simulink library "isi_correlator_lib"  (Simulink 7.3)
settings: Solver=ode45  SolverMode=SingleTasking  StartTime=0.0  StopTime=10.0  RelTol=1e-3
libraries: xbsIndex_r4 x337, casper_library x37, xps_library x31, isi_correlator_lib x28
(part 1 of 3)
settings Model: Creator=wjm  LastModifiedBy=wjm

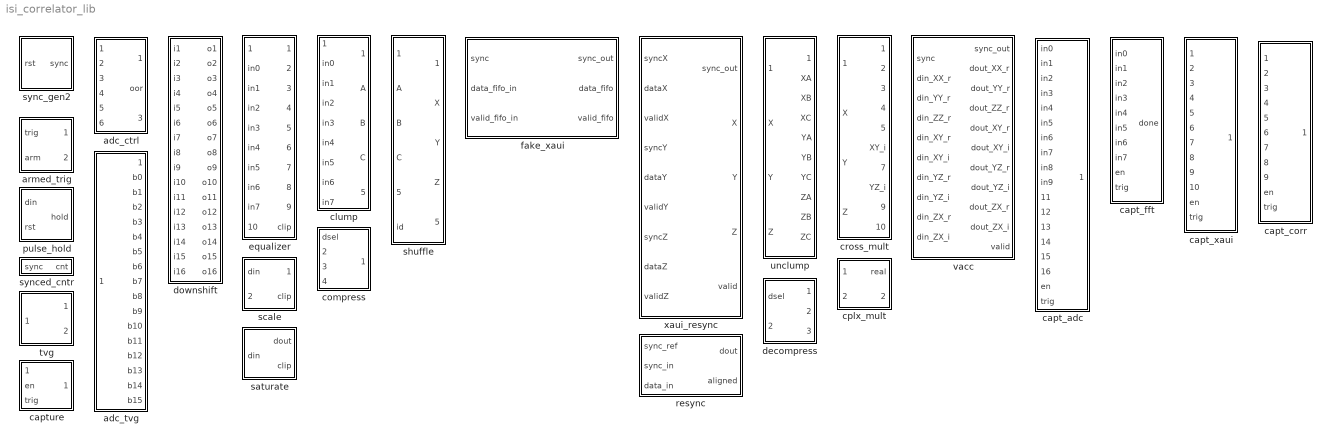
== system isi_correlator_lib ==
  adc_ctrl : Subsystem
  adc_tvg : Subsystem
  armed_trig : Subsystem
  capt_adc : Subsystem
  capt_corr : Subsystem
  capt_fft : Subsystem  mask{bit_width=18}
      mask prompts: bit_width "Bit width:"
  capt_xaui : Subsystem
  capture : Subsystem  mask(capture){num_brams=1, addr_width=11, done_port=off}
      mask prompts: num_brams "Number of BRAMs:"; addr_width "Address width:"; done_port "Provide done port"
      mask help: This block captures N data lines into N separate BRAMs.
      mask init:
      | capture_init(gcb, ...
      |     'num_brams', num_brams, ...
      |     'addr_width', addr_width, ...
      |     'done_port', done_port);
  clump : Subsystem  mask{latency=1}
  compress : Subsystem  mask{latency=1}
  cplx_mult : Subsystem  mask{in_bit_width=4, in_bin_point=3, mult_latency=3, add_latency=2}
      mask prompts: in_bit_width "Input bit width:"; in_bin_point "Input binary point:"; mult_latency "Mult latency:"; add_latency "Add latency:"
  cross_mult : Subsystem  mask{in_bit_width=4, in_bin_point=3, out_bit_width=8, out_bin_point=6, mult_latency=3, add_latency=2}
      mask prompts: in_bit_width "Input bit width: (cplx)"; in_bin_point "Input binary point: (cplx)"; out_bit_width "Output bit width: (cplx)"; out_bin_point "Output binary point: (cplx)"; mult_latency "Mult latency:"; add_latency "Add latency:"
  decompress : Subsystem  mask{latency=1}
  downshift : Subsystem  mask{bit_width=18}
      mask prompts: bit_width "Bit width:"
  equalizer : Subsystem  mask{in_bit_width=18, in_bin_point=17, coeff_bit_width=16, coeff_bin_point=8, out_bit_width=4, out_bin_point=3}
      mask prompts: in_bit_width "Input bit width:"; in_bin_point "Input binary point:"; coeff_bit_width "Coeff bit width:"; coeff_bin_point "Coeff binary point:"; out_bit_width "Output bit width:"; out_bin_point "Output binary point:"
  fake_xaui : Subsystem  mask{latency=64}
  pulse_hold : Subsystem
  resync : Subsystem  mask{depth=4}
      mask prompts: depth "Buffer depth: (2^?)"
  saturate : Subsystem  mask{in_bit_width=34, in_bin_point=25, out_bit_width=4, out_bin_point=3}
      mask prompts: in_bit_width "Input bit width:"; in_bin_point "Input binary point:"; out_bit_width "Output bit width:"; out_bin_point "Output binary point:"
  scale : Subsystem  mask{in_bit_width=8, in_bin_point=7, coeff_bit_width=16, coeff_bin_point=8, out_bit_width=5, out_bin_point=4}
      mask prompts: in_bit_width "Input bit width:"; in_bin_point "Input binary point:"; coeff_bit_width "Coeff bit width:"; coeff_bin_point "Coeff binary point:"; out_bit_width "Output bit width:"; out_bin_point "Output binary point:"
  shuffle : Subsystem  mask{latency=3}
  sync_gen2 : Subsystem  mask(sync_gen2){using_pfb_fir=off, pfb_fir_taps=1, using_fft=on, fft_size=7, fft_inputs=4, fft_orders=1, using_ct=off, ct_type=Double-buffered, using_vacc=off, vacc_length=0, using_scale_factor=off, scale_factor=1}
      mask prompts: using_pfb_fir "This design uses a PFB FIR."; pfb_fir_taps "Number of taps in PFB FIR:"; using_fft "This design uses an FFT."; fft_size "Size of FFT: (2^?)"; fft_inputs "Number of FFT inputs: (2^?)"; fft_orders "Order of FFT reorders: (vector)"; using_ct "This design uses a corner turner."; ct_type "Type of reorder operation:"; using_vacc "This design uses a vector accumulator."; vacc_length "Length of accumulations: (2^?)"; using_scale_factor "Scale the minimum period by an arbitrary amount."; scale_factor "Scale factor:"
      mask help: This block generates a sync pulse of an appropriate period based on the specified mask parameters.
      mask init:
      | sync_gen2_init(gcb, ...
      |     'using_pfb_fir', using_pfb_fir, ...
      |     'pfb_fir_taps', pfb_fir_taps, ...
      |     'using_fft', using_fft, ...
      |     'fft_size', fft_size, ...
      |     'fft_inputs', fft_inputs, ...
      |     'fft_orders', fft_orders, ...
      |     'using_ct', using_ct, ...
      |     'ct_type', ct_type, ...
      |     'using_vacc', using_vacc, ...
      |     'vacc_length', vacc_length, ...
      |     'using_scale_factor', using_scale_factor, ...
      |     'scale_factor', scale_factor);
      settings: AttributesFormatString=sync_period=8
      mask StyleString: checkbox,edit,checkbox,edit,edit,edit,checkbox,popup(Double-buffered|In-place),checkbox,edit,checkbox,edit
      mask CallbackString:
      | thisVariable = 'using_pfb_fir';
      | affectedVars = {'pfb_fir_taps'};
      | 
      | thisBlock = gcb();
      | thisVarState = get_param(thisBlock, thisVariable);
      | maskNames = get_param(thisBlock, 'MaskNames');
      | maskEnables = get_param(thisBlock, 'MaskEnables');
      | 
      | for varName = affectedVars
      |     varIndex = find(ismember(maskNames, varName));
      |     maskEnables{varIndex} = thisVarState;
      | end
      | 
      | set_param(thisBlock, 'MaskEnables', maskEnables);||thisVariable = 'using_fft';
      | affectedVars = {'fft_size', 'fft_inputs', 'fft_orders'};
      | 
      | thisBlock = gcb();
      | thisVarState = get_param(thisBlock, thisVariable);
      | maskNames = get_param(thisBlock, 'MaskNames');
      | maskEnables = get_param(thisBlock, 'MaskEnables');
      | 
      | for varName = affectedVars
      |     varIndex = find(ismember(maskNames, varName));
      |     maskEnables{varIndex} = thisVarState;
      | end
      | 
      | set_param(thisBlock, 'MaskEnables', maskEnables);||||thisVariable = 'using_ct';
      | affectedVars = {'ct_type'};
      | 
      | thisBlock = gcb();
      | thisVarState = get_param(thisBlock, thisVariable);
      | maskNames = get_param(thisBlock, 'MaskNames');
      | maskEnables = get_param(thisBlock, 'MaskEnables');
      | 
      | for varName = affectedVars
      |     varIndex = find(ismember(maskNames, varName));
      |     maskEnables{varIndex} = thisVarState;
      | end
      | 
      | set_param(thisBlock, 'MaskEnables', maskEnables);||thisVariable = 'using_vacc';
      | affectedVars = {'vacc_length'};
      | 
      | thisBlock = gcb();
      | thisVarState = get_param(thisBlock, thisVariable);
      | maskNames = get_param(thisBlock, 'MaskNames');
      | maskEnables = get_param(thisBlock, 'MaskEnables');
      | 
      | for varName = affectedVars
      |     varIndex = find(ismember(maskNames, varName));
      |     maskEnables{varIndex} = thisVarState;
      | end
      | 
      | set_param(thisBlock, 'MaskEnables', maskEnables);||thisVariable = 'using_scale_factor';
      | affectedVars = {'scale_factor'};
      | 
      | thisBlock = gcb();
      | thisVarState = get_param(thisBlock, thisVariable);
      | maskNames = get_param(thisBlock, 'MaskNames');
      | maskEnables = get_param(thisBlock, 'MaskEnables');
      | 
      | for varName = affectedVars
      |     varIndex = find(ismember(maskNames, varName));
      |     maskEnables{varIndex} = thisVarState;
      | end
      | 
      | set_param(thisBlock, 'MaskEnables', maskEnables);|
  synced_cntr : Subsystem  mask{bitwidth=2}
      mask prompts: bitwidth "Counter bitwidth:"
  tvg : Subsystem  mask{addr_width=11}
      mask prompts: addr_width "Address width:"
  unclump : Subsystem  mask{latency=1}
  vacc : Subsystem  mask{vector_length=8, out_bit_width=27, out_bin_point=4, and_delay=2}
      mask prompts: vector_length "Vector length:"; out_bit_width "Output bit width:"; out_bin_point "Output binary point:"; and_delay "Logic delay:"
  xaui_resync : Subsystem  mask(link_demux){buffer_depth=8, logic_latency=1}
      mask prompts: buffer_depth "Buffer depth: (2^n)"; logic_latency "Logic latency:"
      mask help: Demuxes three data streams from five links (one loopback and four xaui). Realigns the streams, and reconstructs a corresponding sync pulse.

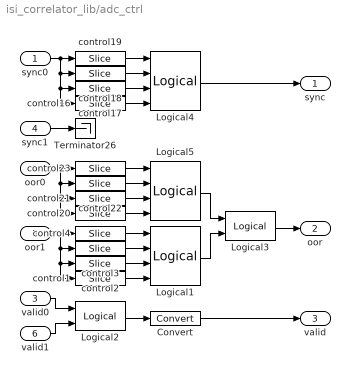
== system isi_correlator_lib/adc_ctrl ==
  sync0 : Inport  OutDataType=sfix(16)  OutScaling=2^0
  oor0 : Inport  Port=2  OutDataType=sfix(16)  OutScaling=2^0
  valid0 : Inport  Port=3  OutDataType=sfix(16)  OutScaling=2^0
  sync1 : Inport  Port=4  OutDataType=sfix(16)  OutScaling=2^0
  oor1 : Inport  Port=5  OutDataType=sfix(16)  OutScaling=2^0
  valid1 : Inport  Port=6  OutDataType=sfix(16)  OutScaling=2^0
  Convert : xbsIndex_r4/Convert  arith_type=Boolean  n_bits=1  bin_pt=0  quantization=Truncate  overflow=Wrap  latency=0  dbl_ovrd=off  pipeline=off  block_type=convert
      settings: block_version=11.3
  Logical1 : xbsIndex_r4/Logical  logical_function=OR  inputs=4  en=off  latency=0  precision=Full  arith_type=Unsigned  n_bits=1  bin_pt=0  align_bp=on  dbl_ovrd=off  block_type=logical
      settings: block_version=10.1.1
  Logical2 : xbsIndex_r4/Logical  logical_function=OR  inputs=2  en=off  latency=0  precision=Full  arith_type=Unsigned  n_bits=1  bin_pt=0  align_bp=on  dbl_ovrd=off  block_type=logical
      settings: block_version=10.1.1
  Logical3 : xbsIndex_r4/Logical  logical_function=OR  inputs=2  en=off  latency=0  precision=Full  arith_type=Unsigned  n_bits=1  bin_pt=0  align_bp=on  dbl_ovrd=off  block_type=logical
      settings: block_version=10.1.1
  Logical4 : xbsIndex_r4/Logical  logical_function=OR  inputs=4  en=off  latency=0  precision=Full  arith_type=Unsigned  n_bits=1  bin_pt=0  align_bp=on  dbl_ovrd=off  block_type=logical
      settings: block_version=10.1.1
  Logical5 : xbsIndex_r4/Logical  logical_function=OR  inputs=4  en=off  latency=0  precision=Full  arith_type=Unsigned  n_bits=1  bin_pt=0  align_bp=on  dbl_ovrd=off  block_type=logical
      settings: block_version=10.1.1
  Terminator26 : Terminator
  control1 : xbsIndex_r4/Slice  nbits=1  boolean_output=on  mode=Lower Bit Location + Width  bit1=0  base1=MSB of Input  bit0=0  base0=LSB of Input  dbl_ovrd=off  block_type=slice
      settings: block_version=10.1.3
  control16 : xbsIndex_r4/Slice  nbits=1  boolean_output=on  mode=Lower Bit Location + Width  bit1=0  base1=MSB of Input  bit0=0  base0=LSB of Input  dbl_ovrd=off  block_type=slice
      settings: block_version=10.1.3
  control17 : xbsIndex_r4/Slice  nbits=1  boolean_output=on  mode=Lower Bit Location + Width  bit1=0  base1=MSB of Input  bit0=1  base0=LSB of Input  dbl_ovrd=off  block_type=slice
      settings: block_version=10.1.3
  control18 : xbsIndex_r4/Slice  nbits=1  boolean_output=on  mode=Lower Bit Location + Width  bit1=0  base1=MSB of Input  bit0=2  base0=LSB of Input  dbl_ovrd=off  block_type=slice
      settings: block_version=10.1.3
  control19 : xbsIndex_r4/Slice  nbits=1  boolean_output=on  mode=Lower Bit Location + Width  bit1=0  base1=MSB of Input  bit0=3  base0=LSB of Input  dbl_ovrd=off  block_type=slice
      settings: block_version=10.1.3
  control2 : xbsIndex_r4/Slice  nbits=1  boolean_output=on  mode=Lower Bit Location + Width  bit1=0  base1=MSB of Input  bit0=1  base0=LSB of Input  dbl_ovrd=off  block_type=slice
      settings: block_version=10.1.3
  control20 : xbsIndex_r4/Slice  nbits=1  boolean_output=on  mode=Lower Bit Location + Width  bit1=0  base1=MSB of Input  bit0=0  base0=LSB of Input  dbl_ovrd=off  block_type=slice
      settings: block_version=10.1.3
  control21 : xbsIndex_r4/Slice  nbits=1  boolean_output=on  mode=Lower Bit Location + Width  bit1=0  base1=MSB of Input  bit0=1  base0=LSB of Input  dbl_ovrd=off  block_type=slice
      settings: block_version=10.1.3
  control22 : xbsIndex_r4/Slice  nbits=1  boolean_output=on  mode=Lower Bit Location + Width  bit1=0  base1=MSB of Input  bit0=2  base0=LSB of Input  dbl_ovrd=off  block_type=slice
      settings: block_version=10.1.3
  control23 : xbsIndex_r4/Slice  nbits=1  boolean_output=on  mode=Lower Bit Location + Width  bit1=0  base1=MSB of Input  bit0=3  base0=LSB of Input  dbl_ovrd=off  block_type=slice
      settings: block_version=10.1.3
  control3 : xbsIndex_r4/Slice  nbits=1  boolean_output=on  mode=Lower Bit Location + Width  bit1=0  base1=MSB of Input  bit0=2  base0=LSB of Input  dbl_ovrd=off  block_type=slice
      settings: block_version=10.1.3
  control4 : xbsIndex_r4/Slice  nbits=1  boolean_output=on  mode=Lower Bit Location + Width  bit1=0  base1=MSB of Input  bit0=3  base0=LSB of Input  dbl_ovrd=off  block_type=slice
      settings: block_version=10.1.3
  sync : Outport  OutDataType=sfix(16)  OutScaling=2^0
  oor : Outport  Port=2  OutDataType=sfix(16)  OutScaling=2^0
  valid : Outport  Port=3  OutDataType=sfix(16)  OutScaling=2^0
  wires:
  Logical2/1 -> Convert/1
  Convert/1 -> valid/1
  control23/1 -> Logical5/1
  control22/1 -> Logical5/2
  control21/1 -> Logical5/3
  control20/1 -> Logical5/4
  sync0/1 -> control19/1, control18/1, control16/1, control17/1
  control19/1 -> Logical4/1
  control18/1 -> Logical4/2
  control17/1 -> Logical4/3
  control16/1 -> Logical4/4
  oor0/1 -> control23/1, control22/1, control20/1, control21/1
  control4/1 -> Logical1/1
  control3/1 -> Logical1/2
  control2/1 -> Logical1/3
  control1/1 -> Logical1/4
  Logical5/1 -> Logical3/1
  Logical1/1 -> Logical3/2
  sync1/1 -> Terminator26/1
  Logical3/1 -> oor/1
  Logical4/1 -> sync/1
  oor1/1 -> control4/1, control3/1, control1/1, control2/1
  valid0/1 -> Logical2/1
  valid1/1 -> Logical2/2

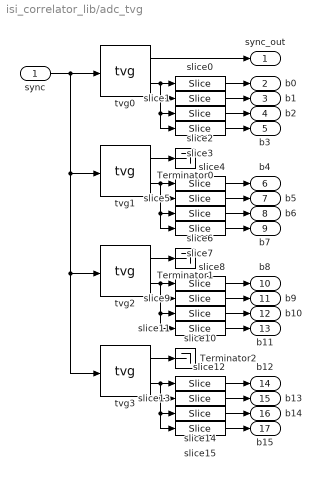
== system isi_correlator_lib/adc_tvg ==
  sync : Inport  OutDataType=sfix(16)  OutScaling=2^0
  Terminator0 : Terminator
  Terminator1 : Terminator
  Terminator2 : Terminator
  slice{0,4,8,12} (4 alike) : xbsIndex_r4/Slice  nbits=8  boolean_output=off  mode=Lower Bit Location + Width  bit1=0  base1=MSB of Input  bit0=0  base0=LSB of Input  dbl_ovrd=off  block_type=slice
      settings: block_version=10.1.3
  slice{1,5,9,13} (4 alike) : xbsIndex_r4/Slice  nbits=8  boolean_output=off  mode=Lower Bit Location + Width  bit1=0  base1=MSB of Input  bit0=8  base0=LSB of Input  dbl_ovrd=off  block_type=slice
      settings: block_version=10.1.3
  slice{2,6,10,14} (4 alike) : xbsIndex_r4/Slice  nbits=8  boolean_output=off  mode=Lower Bit Location + Width  bit1=0  base1=MSB of Input  bit0=16  base0=LSB of Input  dbl_ovrd=off  block_type=slice
      settings: block_version=10.1.3
  slice{3,7,11,15} (4 alike) : xbsIndex_r4/Slice  nbits=8  boolean_output=off  mode=Lower Bit Location + Width  bit1=0  base1=MSB of Input  bit0=24  base0=LSB of Input  dbl_ovrd=off  block_type=slice
      settings: block_version=10.1.3
  tvg{0..3} (4 alike) : isi_correlator_lib/tvg  SystemSampleTime=-1  addr_width=11
  sync_out : Outport
  b0 : Outport  Port=2
  b1 : Outport  Port=3
  b2 : Outport  Port=4
  b3 : Outport  Port=5
  b4 : Outport  Port=6
  b5 : Outport  Port=7
  b6 : Outport  Port=8
  b7 : Outport  Port=9
  b8 : Outport  Port=10
  b9 : Outport  Port=11
  b10 : Outport  Port=12
  b11 : Outport  Port=13
  b12 : Outport  Port=14
  b13 : Outport  Port=15
  b14 : Outport  Port=16
  b15 : Outport  Port=17
  wires:
  tvg3/2 -> slice14/1, slice15/1, slice13/1, slice12/1
  tvg2/2 -> slice10/1, slice11/1, slice9/1, slice8/1
  tvg1/2 -> slice6/1, slice7/1, slice5/1, slice4/1
  tvg0/2 -> slice2/1, slice3/1, slice1/1, slice0/1
  tvg0/1 -> sync_out/1
  slice0/1 -> b0/1
  slice1/1 -> b1/1
  slice2/1 -> b2/1
  slice3/1 -> b3/1
  slice4/1 -> b4/1
  slice5/1 -> b5/1
  slice6/1 -> b6/1
  slice7/1 -> b7/1
  slice8/1 -> b8/1
  slice9/1 -> b9/1
  slice10/1 -> b10/1
  slice11/1 -> b11/1
  slice12/1 -> b12/1
  slice13/1 -> b13/1
  slice14/1 -> b14/1
  slice15/1 -> b15/1
  sync/1 -> tvg0/1, tvg1/1, tvg3/1, tvg2/1
  tvg1/1 -> Terminator0/1
  tvg2/1 -> Terminator1/1
  tvg3/1 -> Terminator2/1

== system isi_correlator_lib/armed_trig ==
  trig : Inport  OutDataType=sfix(16)  OutScaling=2^0
  arm : Inport  Port=2  OutDataType=sfix(16)  OutScaling=2^0
  Constant : xbsIndex_r4/Constant  arith_type=Boolean  const=1  n_bits=1  bin_pt=0  explicit_period=on  period=1  equ=P=C  opselect=C  inp2=PCIN>>17  opr=+  inp1=P  carry=CIN  dbl_ovrd=off  block_type=constant
  Logical : xbsIndex_r4/Logical  logical_function=AND  inputs=2  en=off  latency=0  precision=Full  arith_type=Unsigned  n_bits=16  bin_pt=0  align_bp=on  dbl_ovrd=off  block_type=logical
  Register : xbsIndex_r4/Register  init=0  rst=on  en=on  dbl_ovrd=off  block_type=register
  posedge : casper_library/Misc/posedge  Tag=Rising Edge Detector  SystemSampleTime=-1
  trig_out : Outport  OutDataType=sfix(16)  OutScaling=2^0
  armed : Outport  Port=2  OutDataType=sfix(16)  OutScaling=2^0
  wires:
  trig/1 -> Logical/1
  Register/1 -> Logical/2, armed/1
  arm/1 -> posedge/1
  Constant/1 -> Register/1
  posedge/1 -> Register/3
  Logical/1 -> trig_out/1, Register/2

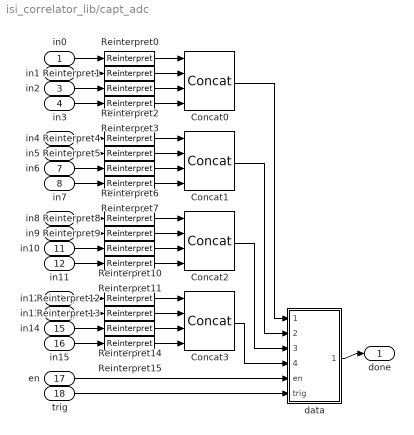
== system isi_correlator_lib/capt_adc ==
  in0 : Inport
  in1 : Inport  Port=2
  in2 : Inport  Port=3
  in3 : Inport  Port=4
  in4 : Inport  Port=5
  in5 : Inport  Port=6
  in6 : Inport  Port=7
  in7 : Inport  Port=8
  in8 : Inport  Port=9
  in9 : Inport  Port=10
  in10 : Inport  Port=11
  in11 : Inport  Port=12
  in12 : Inport  Port=13
  in13 : Inport  Port=14
  in14 : Inport  Port=15
  in15 : Inport  Port=16
  en : Inport  Port=17
  trig : Inport  Port=18
  Concat{0..3} (4 alike) : xbsIndex_r4/Concat  num_inputs=4  dbl_ovrd=off  block_type=concat
      settings: block_version=10.1.3
  Reinterpret{0..15} (16 alike) : xbsIndex_r4/Reinterpret  force_arith_type=on  arith_type=Unsigned  force_bin_pt=on  bin_pt=0  block_type=reinterpret
      settings: infoedit="Changes signal type without altering the binary representation.   You can changed the signal between signed and unsigned, and relocate the binary point.<P><P>Hardware notes: In hardware this block costs nothing.<P><P>Example:  Suppose the input is 6 bits wide, signed, with 2 fractional bits, and the output is forced to unsigned with 0 fractional bits.  Then an input of -2.0 (1110.00 in binary 2's complement) becomes an output of 56 (111000 in binary)."  block_version=10.1.3
  data : Subsystem  AncestorBlock=isi_correlator_lib/capture  mask(capture){num_brams=4, addr_width=11, done_port=on}
      mask prompts: num_brams "Number of BRAMs:"; addr_width "Address width:"; done_port "Provide done port"
      mask help: This block captures N data lines into N separate BRAMs.
      mask init:
      | capture_init(gcb, ...
      |     'num_brams', num_brams, ...
      |     'addr_width', addr_width, ...
      |     'done_port', done_port);
  done : Outport
  wires:
  Concat3/1 -> data/4(din3)
  Concat2/1 -> data/3(din2)
  Concat1/1 -> data/2(din1)
  Concat0/1 -> data/1(din0)
  trig/1 -> data/6(trig)
  en/1 -> data/5(en)
  Reinterpret15/1 -> Concat3/4
  Reinterpret14/1 -> Concat3/3
  Reinterpret13/1 -> Concat3/2
  Reinterpret12/1 -> Concat3/1
  Reinterpret11/1 -> Concat2/4
  Reinterpret10/1 -> Concat2/3
  Reinterpret9/1 -> Concat2/2
  Reinterpret8/1 -> Concat2/1
  Reinterpret7/1 -> Concat1/4
  Reinterpret6/1 -> Concat1/3
  Reinterpret5/1 -> Concat1/2
  Reinterpret4/1 -> Concat1/1
  Reinterpret3/1 -> Concat0/4
  Reinterpret2/1 -> Concat0/3
  Reinterpret1/1 -> Concat0/2
  Reinterpret0/1 -> Concat0/1
  in0/1 -> Reinterpret0/1
  in1/1 -> Reinterpret1/1
  in2/1 -> Reinterpret2/1
  in3/1 -> Reinterpret3/1
  in4/1 -> Reinterpret4/1
  in5/1 -> Reinterpret5/1
  in6/1 -> Reinterpret6/1
  in7/1 -> Reinterpret7/1
  in8/1 -> Reinterpret8/1
  in9/1 -> Reinterpret9/1
  in10/1 -> Reinterpret10/1
  in11/1 -> Reinterpret11/1
  in12/1 -> Reinterpret12/1
  in13/1 -> Reinterpret13/1
  in14/1 -> Reinterpret14/1
  in15/1 -> Reinterpret15/1
  data/1(done) -> done/1

== system isi_correlator_lib/capt_corr ==
  AA_r : Inport
  BB_r : Inport  Port=2
  CC_r : Inport  Port=3
  AB_r : Inport  Port=4
  AB_i : Inport  Port=5
  BC_r : Inport  Port=6
  BC_i : Inport  Port=7
  CA_r : Inport  Port=8
  CA_i : Inport  Port=9
  en : Inport  Port=10
  trig : Inport  Port=11
  capt0 : Subsystem  AncestorBlock=isi_correlator_lib/capture  mask(capture){num_brams=3, addr_width=11, done_port=off}
      mask prompts: num_brams "Number of BRAMs:"; addr_width "Address width:"; done_port "Provide done port"
      mask help: This block captures N data lines into N separate BRAMs.
      mask init:
      | capture_init(gcb, ...
      |     'num_brams', num_brams, ...
      |     'addr_width', addr_width, ...
      |     'done_port', done_port);
  capt1 : Subsystem  AncestorBlock=isi_correlator_lib/capture  mask(capture){num_brams=3, addr_width=11, done_port=off}
      mask prompts: num_brams "Number of BRAMs:"; addr_width "Address width:"; done_port "Provide done port"
      mask help: This block captures N data lines into N separate BRAMs.
      mask init:
      | capture_init(gcb, ...
      |     'num_brams', num_brams, ...
      |     'addr_width', addr_width, ...
      |     'done_port', done_port);
  capt2 : Subsystem  AncestorBlock=isi_correlator_lib/capture  mask(capture){num_brams=3, addr_width=11, done_port=off}
      mask prompts: num_brams "Number of BRAMs:"; addr_width "Address width:"; done_port "Provide done port"
      mask help: This block captures N data lines into N separate BRAMs.
      mask init:
      | capture_init(gcb, ...
      |     'num_brams', num_brams, ...
      |     'addr_width', addr_width, ...
      |     'done_port', done_port);
  done : Outport
  wires:
  AA_r/1 -> capt0/1(din0)
  BB_r/1 -> capt0/2(din1)
  CC_r/1 -> capt0/3(din2)
  AB_r/1 -> capt1/1(din0)
  AB_i/1 -> capt1/2(din1)
  BC_r/1 -> capt1/3(din2)
  BC_i/1 -> capt2/1(din0)
  CA_r/1 -> capt2/2(din1)
  CA_i/1 -> capt2/3(din2)
  en/1 -> capt2/4(en), capt0/4(en), capt1/4(en)
  trig/1 -> capt2/5(trig), capt0/5(trig), capt1/5(trig)
  capt0/1(done) -> done/1

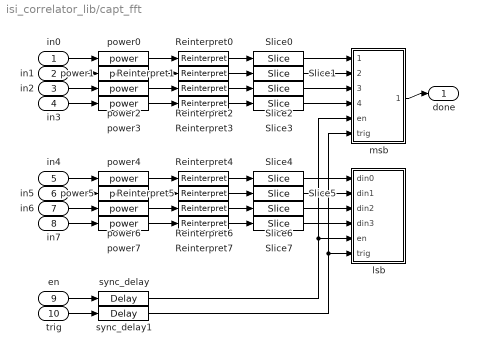
== system isi_correlator_lib/capt_fft ==
  in0 : Inport
  in1 : Inport  Port=2
  in2 : Inport  Port=3
  in3 : Inport  Port=4
  in4 : Inport  Port=5
  in5 : Inport  Port=6
  in6 : Inport  Port=7
  in7 : Inport  Port=8
  en : Inport  Port=9
  trig : Inport  Port=10
  Reinterpret{0..7} (8 alike) : xbsIndex_r4/Reinterpret  force_arith_type=on  arith_type=Unsigned  force_bin_pt=on  bin_pt=0  block_type=reinterpret
      settings: infoedit="Changes signal type without altering the binary representation.   You can changed the signal between signed and unsigned, and relocate the binary point.<P><P>Hardware notes: In hardware this block costs nothing.<P><P>Example:  Suppose the input is 6 bits wide, signed, with 2 fractional bits, and the output is forced to unsigned with 0 fractional bits.  Then an input of -2.0 (1110.00 in binary 2's complement) becomes an output of 56 (111000 in binary)."  block_version=10.1.3
  Slice{0..7} (8 alike) : xbsIndex_r4/Slice  nbits=min(32, bit_width*2)  boolean_output=off  mode=Upper Bit Location + Width  bit1=0  base1=MSB of Input  bit0=0  base0=LSB of Input  dbl_ovrd=off  block_type=slice
      settings: block_version=11.3
  lsb : Subsystem  AncestorBlock=isi_correlator_lib/capture  mask(capture){num_brams=4, addr_width=11, done_port=off}
      mask prompts: num_brams "Number of BRAMs:"; addr_width "Address width:"; done_port "Provide done port"
      mask help: This block captures N data lines into N separate BRAMs.
      mask init:
      | capture_init(gcb, ...
      |     'num_brams', num_brams, ...
      |     'addr_width', addr_width, ...
      |     'done_port', done_port);
  msb : Subsystem  AncestorBlock=isi_correlator_lib/capture  mask(capture){num_brams=4, addr_width=11, done_port=off}
      mask prompts: num_brams "Number of BRAMs:"; addr_width "Address width:"; done_port "Provide done port"
      mask help: This block captures N data lines into N separate BRAMs.
      mask init:
      | capture_init(gcb, ...
      |     'num_brams', num_brams, ...
      |     'addr_width', addr_width, ...
      |     'done_port', done_port);
  power{0..7} (8 alike) : casper_library/Misc/power  SystemSampleTime=-1  BitWidth=bit_width  add_latency=2  mult_latency=3
  sync_delay : xbsIndex_r4/Delay  en=off  latency=5  dbl_ovrd=off  reg_retiming=off  block_type=delay
  sync_delay1 : xbsIndex_r4/Delay  en=off  latency=5  dbl_ovrd=off  reg_retiming=off  block_type=delay
  done : Outport
  wires:
  power7/1 -> Reinterpret7/1
  in7/1 -> power7/1
  trig/1 -> sync_delay1/1
  en/1 -> sync_delay/1
  Reinterpret3/1 -> Slice3/1
  Reinterpret2/1 -> Slice2/1
  Reinterpret1/1 -> Slice1/1
  Reinterpret7/1 -> Slice7/1
  Reinterpret6/1 -> Slice6/1
  Reinterpret5/1 -> Slice5/1
  Reinterpret4/1 -> Slice4/1
  power6/1 -> Reinterpret6/1
  in6/1 -> power6/1
  power5/1 -> Reinterpret5/1
  in5/1 -> power5/1
  power4/1 -> Reinterpret4/1
  in4/1 -> power4/1
  power3/1 -> Reinterpret3/1
  in3/1 -> power3/1
  power2/1 -> Reinterpret2/1
  in2/1 -> power2/1
  power1/1 -> Reinterpret1/1
  in1/1 -> power1/1
  Reinterpret0/1 -> Slice0/1
  power0/1 -> Reinterpret0/1
  in0/1 -> power0/1
  sync_delay/1 -> msb/5(en), lsb/5(en)
  sync_delay1/1 -> msb/6(trig), lsb/6(trig)
  Slice0/1 -> msb/1(din0)
  Slice1/1 -> msb/2(din1)
  Slice2/1 -> msb/3(din2)
  Slice3/1 -> msb/4(din3)
  Slice4/1 -> lsb/1(din0)
  Slice5/1 -> lsb/2(din1)
  Slice6/1 -> lsb/3(din2)
  Slice7/1 -> lsb/4(din3)
  msb/1(done) -> done/1

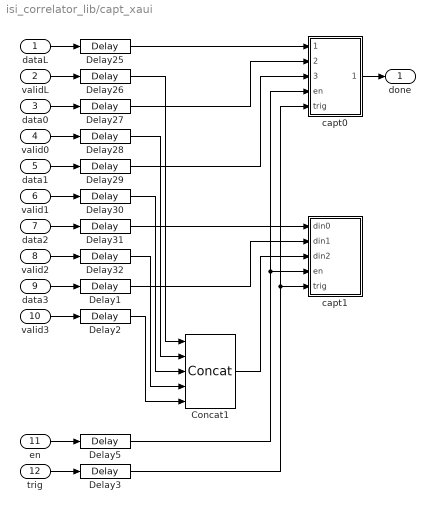
== system isi_correlator_lib/capt_xaui ==
  dataL : Inport
  validL : Inport  Port=2
  data0 : Inport  Port=3
  valid0 : Inport  Port=4
  data1 : Inport  Port=5
  valid1 : Inport  Port=6
  data2 : Inport  Port=7
  valid2 : Inport  Port=8
  data3 : Inport  Port=9
  valid3 : Inport  Port=10
  en : Inport  Port=11
  trig : Inport  Port=12
  Concat1 : xbsIndex_r4/Concat  num_inputs=5  dbl_ovrd=off  block_type=concat
      settings: block_version=10.1.3
  Delay{1..3,5,25..32} (12 alike) : xbsIndex_r4/Delay  en=off  latency=2  dbl_ovrd=off  reg_retiming=off  block_type=delay
  capt0 : Subsystem  AncestorBlock=isi_correlator_lib/capture  mask(capture){num_brams=3, addr_width=11, done_port=off}
      mask prompts: num_brams "Number of BRAMs:"; addr_width "Address width:"; done_port "Provide done port"
      mask help: This block captures N data lines into N separate BRAMs.
      mask init:
      | capture_init(gcb, ...
      |     'num_brams', num_brams, ...
      |     'addr_width', addr_width, ...
      |     'done_port', done_port);
  capt1 : Subsystem  AncestorBlock=isi_correlator_lib/capture  mask(capture){num_brams=3, addr_width=11, done_port=off}
      mask prompts: num_brams "Number of BRAMs:"; addr_width "Address width:"; done_port "Provide done port"
      mask help: This block captures N data lines into N separate BRAMs.
      mask init:
      | capture_init(gcb, ...
      |     'num_brams', num_brams, ...
      |     'addr_width', addr_width, ...
      |     'done_port', done_port);
  done : Outport
  wires:
  dataL/1 -> Delay25/1
  validL/1 -> Delay26/1
  data0/1 -> Delay27/1
  valid0/1 -> Delay28/1
  data1/1 -> Delay29/1
  valid1/1 -> Delay30/1
  data2/1 -> Delay31/1
  valid2/1 -> Delay32/1
  data3/1 -> Delay1/1
  valid3/1 -> Delay2/1
  Delay26/1 -> Concat1/1
  Delay28/1 -> Concat1/2
  Delay30/1 -> Concat1/3
  Delay32/1 -> Concat1/4
  Delay2/1 -> Concat1/5
  Delay31/1 -> capt1/1(din0)
  Delay1/1 -> capt1/2(din1)
  Concat1/1 -> capt1/3(din2)
  Delay25/1 -> capt0/1(din0)
  Delay27/1 -> capt0/2(din1)
  Delay29/1 -> capt0/3(din2)
  en/1 -> Delay5/1
  trig/1 -> Delay3/1
  Delay5/1 -> capt0/4(en), capt1/4(en)
  Delay3/1 -> capt0/5(trig), capt1/5(trig)
  capt0/1(done) -> done/1

== system isi_correlator_lib/capture ==
  din0 : Inport
  en : Inport  Port=2
  trig : Inport  Port=3
  Constant : xbsIndex_r4/Constant  arith_type=Boolean  const=1  n_bits=1  bin_pt=0  explicit_period=on  period=1  equ=P=C  opselect=C  inp2=PCIN>>17  opr=+  inp1=P  carry=CIN  dbl_ovrd=off  block_type=constant
      settings: block_version=11.3
  Logical : xbsIndex_r4/Logical  logical_function=AND  inputs=2  en=off  latency=0  precision=Full  arith_type=Unsigned  n_bits=16  bin_pt=0  align_bp=on  dbl_ovrd=off  block_type=logical
      settings: block_version=11.3
  bram0 : xps_library/Shared BRAM  Tag=xps:bram  SystemSampleTime=-1  arith_type=Unsigned  addr_width=addr_width  data_width=32  data_bin_pt=0  init_vals=0  sample_rate=1
  freeze_cntr : casper_library/Misc/freeze_cntr  SystemSampleTime=-1  CounterBits=addr_width
  reinterp0 : xbsIndex_r4/Reinterpret  force_arith_type=on  arith_type=Unsigned  force_bin_pt=on  bin_pt=0  block_type=reinterpret
      settings: infoedit="Changes signal type without altering the binary representation.   You can changed the signal between signed and unsigned, and relocate the binary point.<br><br>Hardware notes: In hardware this block costs nothing.<br><br>Example:  Suppose the input is 6 bits wide, signed, with 2 fractional bits, and the output is forced to unsigned with 0 fractional bits.  Then an input of -2.0 (1110.00 in binary 2's complement) becomes an output of 56 (111000 in binary)."  block_version=11.3
  terminator0 : Terminator
  done : Outport
  wires:
  din0/1 -> reinterp0/1
  reinterp0/1 -> bram0/2
  bram0/1 -> terminator0/1
  freeze_cntr/3 -> done/1
  en/1 -> Logical/1
  trig/1 -> Logical/2
  Constant/1 -> freeze_cntr/1
  Logical/1 -> freeze_cntr/2
  freeze_cntr/1 -> bram0/1
  freeze_cntr/2 -> bram0/3

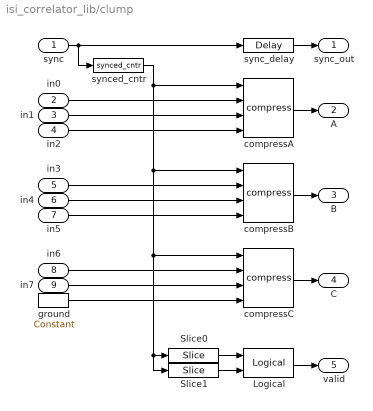
== system isi_correlator_lib/clump ==
  sync : Inport
  in0 : Inport  Port=2
  in1 : Inport  Port=3
  in2 : Inport  Port=4
  in3 : Inport  Port=5
  in4 : Inport  Port=6
  in5 : Inport  Port=7
  in6 : Inport  Port=8
  in7 : Inport  Port=9
  Logical : xbsIndex_r4/Logical  logical_function=OR  inputs=2  en=off  latency=latency  precision=Full  arith_type=Unsigned  n_bits=16  bin_pt=0  align_bp=on  dbl_ovrd=off  block_type=logical
  Slice0 : xbsIndex_r4/Slice  nbits=1  boolean_output=on  mode=Lower Bit Location + Width  bit1=0  base1=MSB of Input  bit0=0  base0=LSB of Input  dbl_ovrd=off  block_type=slice
      settings: block_version=10.1.1
  Slice1 : xbsIndex_r4/Slice  nbits=1  boolean_output=on  mode=Lower Bit Location + Width  bit1=0  base1=MSB of Input  bit0=1  base0=LSB of Input  dbl_ovrd=off  block_type=slice
      settings: block_version=10.1.1
  compressA : isi_correlator_lib/compress  SystemSampleTime=-1  latency=latency
  compressB : isi_correlator_lib/compress  SystemSampleTime=-1  latency=latency
  compressC : isi_correlator_lib/compress  SystemSampleTime=-1  latency=latency
  ground : xbsIndex_r4/Constant  arith_type=Unsigned  const=0  n_bits=8  bin_pt=0  explicit_period=on  period=1  equ=P=C  opselect=C  inp2=PCIN>>17  opr=+  inp1=P  carry=CIN  dbl_ovrd=off  block_type=constant
      settings: block_version=10.1.1
  sync_delay : xbsIndex_r4/Delay  en=off  latency=latency  dbl_ovrd=off  reg_retiming=off  block_type=delay
  synced_cntr : isi_correlator_lib/synced_cntr  SystemSampleTime=-1  bitwidth=2
  sync_out : Outport
  A : Outport  Port=2
  B : Outport  Port=3
  C : Outport  Port=4
  valid : Outport  Port=5
  wires:
  Slice0/1 -> Logical/1
  Slice1/1 -> Logical/2
  Logical/1 -> valid/1
  compressA/1 -> A/1
  compressB/1 -> B/1
  compressC/1 -> C/1
  sync_delay/1 -> sync_out/1
  sync/1 -> sync_delay/1, synced_cntr/1
  in3/1 -> compressB/2
  in4/1 -> compressB/3
  in5/1 -> compressB/4
  in6/1 -> compressC/2
  in7/1 -> compressC/3
  ground/1 -> compressC/4
  in0/1 -> compressA/2
  in1/1 -> compressA/3
  in2/1 -> compressA/4
  synced_cntr/1 -> Slice1/1, Slice0/1, compressC/1, compressB/1, compressA/1

== system isi_correlator_lib/compress ==
  dsel : Inport
  din0 : Inport  Port=2
  din1 : Inport  Port=3
  din2 : Inport  Port=4
  Concat0 : xbsIndex_r4/Concat  num_inputs=3  dbl_ovrd=off  block_type=concat
      settings: block_version=11.3
  Concat1 : xbsIndex_r4/Concat  num_inputs=2  dbl_ovrd=off  block_type=concat
      settings: block_version=11.3
  Constant : xbsIndex_r4/Constant  arith_type=Unsigned  const=0  n_bits=32  bin_pt=0  explicit_period=on  period=1  equ=P=C  opselect=C  inp2=PCIN>>17  opr=+  inp1=P  carry=CIN  dbl_ovrd=off  block_type=constant
      settings: block_version=11.3
  Delay0 : xbsIndex_r4/Delay  en=off  latency=1  dbl_ovrd=off  reg_retiming=off  block_type=delay
  Mux : xbsIndex_r4/Mux  inputs=4  en=off  latency=latency  precision=Full  arith_type=Unsigned  n_bits=16  bin_pt=14  quantization=Truncate  overflow=Wrap  dbl_ovrd=off  block_type=mux
  Slice0 : xbsIndex_r4/Slice  nbits=32  boolean_output=off  mode=Upper Bit Location + Width  bit1=0  base1=MSB of Input  bit0=0  base0=LSB of Input  dbl_ovrd=off  block_type=slice
      settings: block_version=10.1.1
  Slice1 : xbsIndex_r4/Slice  nbits=32  boolean_output=off  mode=Upper Bit Location + Width  bit1=-8  base1=MSB of Input  bit0=0  base0=LSB of Input  dbl_ovrd=off  block_type=slice
      settings: block_version=10.1.1
  Slice2 : xbsIndex_r4/Slice  nbits=32  boolean_output=off  mode=Upper Bit Location + Width  bit1=-16  base1=MSB of Input  bit0=0  base0=LSB of Input  dbl_ovrd=off  block_type=slice
      settings: block_version=10.1.1
  data : Outport
  wires:
  din0/1 -> Concat0/1
  din1/1 -> Concat0/2
  din2/1 -> Concat0/3
  Concat0/1 -> Delay0/1, Concat1/2
  Delay0/1 -> Concat1/1
  Concat1/1 -> Slice0/1, Slice2/1, Slice1/1
  dsel/1 -> Mux/1
  Mux/1 -> data/1
  Constant/1 -> Mux/2
  Slice0/1 -> Mux/3
  Slice1/1 -> Mux/4
  Slice2/1 -> Mux/5

== system isi_correlator_lib/cplx_mult ==
  a+bi : Inport  OutDataType=sfix(16)  OutScaling=2^0
  c+di : Inport  Port=2  OutDataType=sfix(16)  OutScaling=2^0
  c_to_ri : casper_library/Misc/c_to_ri  SystemSampleTime=-1  n_bits=in_bit_width  bin_pt=in_bin_point
      settings: AttributesFormatString=_ r/i
  c_to_ri1 : casper_library/Misc/c_to_ri  SystemSampleTime=-1  n_bits=in_bit_width  bin_pt=in_bin_point
      settings: AttributesFormatString=_ r/i
  cmult_4bit_em* : casper_library/Multipliers/cmult_4bit_em*  SystemSampleTime=-1  mult_latency=mult_latency  add_latency=add_latency
  real : Outport  OutDataType=sfix(16)  OutScaling=2^0
  imag : Outport  Port=2  OutDataType=sfix(16)  OutScaling=2^0
  wires:
  c_to_ri/1 -> cmult_4bit_em*/1
  c_to_ri/2 -> cmult_4bit_em*/2
  c_to_ri1/1 -> cmult_4bit_em*/3
  c_to_ri1/2 -> cmult_4bit_em*/4
  a+bi/1 -> c_to_ri/1
  c+di/1 -> c_to_ri1/1
  cmult_4bit_em*/1 -> real/1
  cmult_4bit_em*/2 -> imag/1

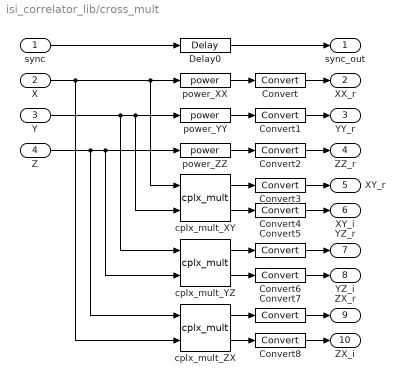
== system isi_correlator_lib/cross_mult ==
  sync : Inport  OutDataType=sfix(16)  OutScaling=2^0
  X : Inport  Port=2  OutDataType=sfix(16)  OutScaling=2^0
  Y : Inport  Port=3  OutDataType=sfix(16)  OutScaling=2^0
  Z : Inport  Port=4  OutDataType=sfix(16)  OutScaling=2^0
  Convert{,1..8} (9 alike) : xbsIndex_r4/Convert  arith_type="Signed  (2's comp)"  n_bits=out_bit_width  bin_pt=out_bin_point  quantization=Truncate  overflow=Wrap  latency=0  dbl_ovrd=off  pipeline=off  block_type=convert
      settings: block_version=10.1.3
  Delay0 : xbsIndex_r4/Delay  en=off  latency=mult_latency + add_latency  dbl_ovrd=off  reg_retiming=off  block_type=delay
  cplx_mult_XY : isi_correlator_lib/cplx_mult  SystemSampleTime=-1  in_bit_width=in_bit_width  in_bin_point=in_bin_point  mult_latency=mult_latency  add_latency=add_latency
  cplx_mult_YZ : isi_correlator_lib/cplx_mult  SystemSampleTime=-1  in_bit_width=in_bit_width  in_bin_point=in_bin_point  mult_latency=mult_latency  add_latency=add_latency
  cplx_mult_ZX : isi_correlator_lib/cplx_mult  SystemSampleTime=-1  in_bit_width=in_bit_width  in_bin_point=in_bin_point  mult_latency=mult_latency  add_latency=add_latency
  power_XX : casper_library/Misc/power  SystemSampleTime=-1  BitWidth=in_bit_width  add_latency=add_latency  mult_latency=mult_latency
  power_YY : casper_library/Misc/power  SystemSampleTime=-1  BitWidth=in_bit_width  add_latency=add_latency  mult_latency=mult_latency
  power_ZZ : casper_library/Misc/power  SystemSampleTime=-1  BitWidth=in_bit_width  add_latency=add_latency  mult_latency=mult_latency
  sync_out : Outport  OutDataType=sfix(16)  OutScaling=2^0
  XX_r : Outport  Port=2  OutDataType=sfix(16)  OutScaling=2^0
  YY_r : Outport  Port=3  OutDataType=sfix(16)  OutScaling=2^0
  ZZ_r : Outport  Port=4  OutDataType=sfix(16)  OutScaling=2^0
  XY_r : Outport  Port=5  OutDataType=sfix(16)  OutScaling=2^0
  XY_i : Outport  Port=6  OutDataType=sfix(16)  OutScaling=2^0
  YZ_r : Outport  Port=7  OutDataType=sfix(16)  OutScaling=2^0
  YZ_i : Outport  Port=8  OutDataType=sfix(16)  OutScaling=2^0
  ZX_r : Outport  Port=9  OutDataType=sfix(16)  OutScaling=2^0
  ZX_i : Outport  Port=10  OutDataType=sfix(16)  OutScaling=2^0
  wires:
  Convert8/1 -> ZX_i/1
  Convert7/1 -> ZX_r/1
  Convert6/1 -> YZ_i/1
  Convert5/1 -> YZ_r/1
  Convert4/1 -> XY_i/1
  Convert3/1 -> XY_r/1
  Convert2/1 -> ZZ_r/1
  Convert1/1 -> YY_r/1
  Convert/1 -> XX_r/1
  cplx_mult_ZX/2 -> Convert8/1
  cplx_mult_ZX/1 -> Convert7/1
  cplx_mult_YZ/2 -> Convert6/1
  cplx_mult_YZ/1 -> Convert5/1
  cplx_mult_XY/2 -> Convert4/1
  cplx_mult_XY/1 -> Convert3/1
  power_ZZ/1 -> Convert2/1
  power_YY/1 -> Convert1/1
  power_XX/1 -> Convert/1
  X/1 -> cplx_mult_XY/1, power_XX/1, cplx_mult_ZX/2
  Y/1 -> cplx_mult_XY/2, power_YY/1, cplx_mult_YZ/1
  Z/1 -> cplx_mult_YZ/2, power_ZZ/1, cplx_mult_ZX/1
  Delay0/1 -> sync_out/1
  sync/1 -> Delay0/1

== system isi_correlator_lib/decompress ==
  dsel : Inport
  data : Inport  Port=2
  Concat1 : xbsIndex_r4/Concat  num_inputs=2  dbl_ovrd=off  block_type=concat
      settings: block_version=11.3
  Delay0 : xbsIndex_r4/Delay  en=off  latency=1  dbl_ovrd=off  reg_retiming=off  block_type=delay
  Mux : xbsIndex_r4/Mux  inputs=4  en=off  latency=latency  precision=Full  arith_type=Unsigned  n_bits=16  bin_pt=14  quantization=Truncate  overflow=Wrap  dbl_ovrd=off  block_type=mux
  Slice0 : xbsIndex_r4/Slice  nbits=24  boolean_output=off  mode=Lower Bit Location + Width  bit1=0  base1=MSB of Input  bit0=8  base0=LSB of Input  dbl_ovrd=off  block_type=slice
      settings: block_version=10.1.1
  Slice1 : xbsIndex_r4/Slice  nbits=24  boolean_output=off  mode=Lower Bit Location + Width  bit1=0  base1=MSB of Input  bit0=16  base0=LSB of Input  dbl_ovrd=off  block_type=slice
      settings: block_version=10.1.1
  Slice2 : xbsIndex_r4/Slice  nbits=24  boolean_output=off  mode=Lower Bit Location + Width  bit1=0  base1=MSB of Input  bit0=24  base0=LSB of Input  dbl_ovrd=off  block_type=slice
      settings: block_version=10.1.1
  Slice3 : xbsIndex_r4/Slice  nbits=24  boolean_output=off  mode=Lower Bit Location + Width  bit1=0  base1=MSB of Input  bit0=32  base0=LSB of Input  dbl_ovrd=off  block_type=slice
      settings: block_version=10.1.1
  Slice4 : xbsIndex_r4/Slice  nbits=8  boolean_output=off  mode=Upper Bit Location + Width  bit1=0  base1=MSB of Input  bit0=0  base0=LSB of Input  dbl_ovrd=off  block_type=slice
      settings: block_version=10.1.1
  Slice5 : xbsIndex_r4/Slice  nbits=8  boolean_output=off  mode=Upper Bit Location + Width  bit1=-8  base1=MSB of Input  bit0=0  base0=LSB of Input  dbl_ovrd=off  block_type=slice
      settings: block_version=10.1.1
  Slice6 : xbsIndex_r4/Slice  nbits=8  boolean_output=off  mode=Upper Bit Location + Width  bit1=-16  base1=MSB of Input  bit0=0  base0=LSB of Input  dbl_ovrd=off  block_type=slice
      settings: block_version=10.1.1
  dout0 : Outport
  dout1 : Outport  Port=2
  dout2 : Outport  Port=3
  wires:
  Concat1/1 -> Slice0/1, Slice1/1, Slice3/1, Slice2/1
  Slice0/1 -> Mux/2
  Slice1/1 -> Mux/3
  Slice2/1 -> Mux/4
  Slice3/1 -> Mux/5
  dsel/1 -> Mux/1
  Mux/1 -> Slice4/1, Slice5/1, Slice6/1
  Delay0/1 -> Concat1/1
  data/1 -> Delay0/1, Concat1/2
  Slice4/1 -> dout0/1
  Slice5/1 -> dout1/1
  Slice6/1 -> dout2/1

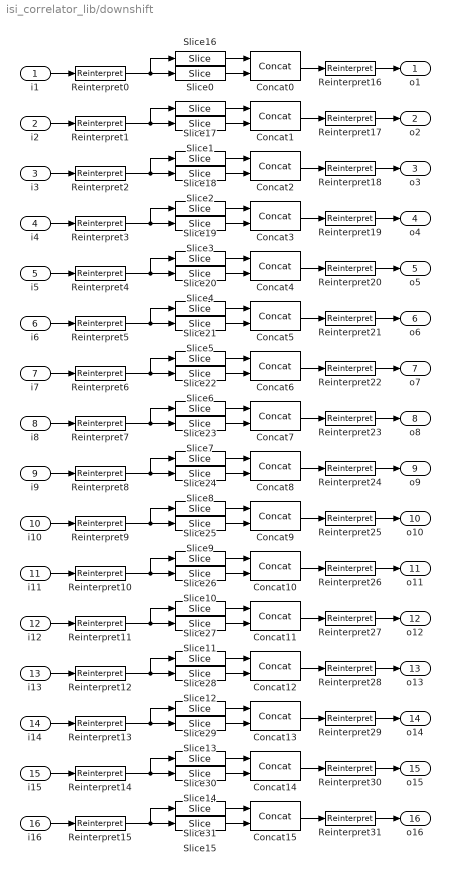
== system isi_correlator_lib/downshift ==
  i1 : Inport
  i2 : Inport  Port=2
  i3 : Inport  Port=3
  i4 : Inport  Port=4
  i5 : Inport  Port=5
  i6 : Inport  Port=6
  i7 : Inport  Port=7
  i8 : Inport  Port=8
  i9 : Inport  Port=9
  i10 : Inport  Port=10
  i11 : Inport  Port=11
  i12 : Inport  Port=12
  i13 : Inport  Port=13
  i14 : Inport  Port=14
  i15 : Inport  Port=15
  i16 : Inport  Port=16
  Concat{0..15} (16 alike) : xbsIndex_r4/Concat  num_inputs=2  dbl_ovrd=off  block_type=concat
      settings: block_version=11.3
  Reinterpret{0..15} (16 alike) : xbsIndex_r4/Reinterpret  force_arith_type=on  arith_type=Unsigned  force_bin_pt=on  bin_pt=0  block_type=reinterpret
      settings: infoedit="Changes signal type without altering the binary representation.   You can changed the signal between signed and unsigned, and relocate the binary point.<br><br>Hardware notes: In hardware this block costs nothing.<br><br>Example:  Suppose the input is 6 bits wide, signed, with 2 fractional bits, and the output is forced to unsigned with 0 fractional bits.  Then an input of -2.0 (1110.00 in binary 2's complement) becomes an output of 56 (111000 in binary)."  block_version=11.3
  Reinterpret{16..31} (16 alike) : xbsIndex_r4/Reinterpret  force_arith_type=on  arith_type="Signed  (2's comp)"  force_bin_pt=on  bin_pt=bit_width - 1  block_type=reinterpret
      settings: infoedit="Changes signal type without altering the binary representation.   You can changed the signal between signed and unsigned, and relocate the binary point.<br><br>Hardware notes: In hardware this block costs nothing.<br><br>Example:  Suppose the input is 6 bits wide, signed, with 2 fractional bits, and the output is forced to unsigned with 0 fractional bits.  Then an input of -2.0 (1110.00 in binary 2's complement) becomes an output of 56 (111000 in binary)."  block_version=11.3
  Slice{0..15} (16 alike) : xbsIndex_r4/Slice  nbits=bit_width - 1  boolean_output=off  mode=Upper Bit Location + Width  bit1=0  base1=MSB of Input  bit0=0  base0=LSB of Input  dbl_ovrd=off  block_type=slice
      settings: block_version=11.3
  Slice{16..31} (16 alike) : xbsIndex_r4/Slice  nbits=1  boolean_output=off  mode=Upper Bit Location + Width  bit1=0  base1=MSB of Input  bit0=0  base0=LSB of Input  dbl_ovrd=off  block_type=slice
      settings: block_version=11.3
  o1 : Outport
  o2 : Outport  Port=2
  o3 : Outport  Port=3
  o4 : Outport  Port=4
  o5 : Outport  Port=5
  o6 : Outport  Port=6
  o7 : Outport  Port=7
  o8 : Outport  Port=8
  o9 : Outport  Port=9
  o10 : Outport  Port=10
  o11 : Outport  Port=11
  o12 : Outport  Port=12
  o13 : Outport  Port=13
  o14 : Outport  Port=14
  o15 : Outport  Port=15
  o16 : Outport  Port=16
  wires:
  Reinterpret31/1 -> o16/1
  Reinterpret30/1 -> o15/1
  Reinterpret29/1 -> o14/1
  Reinterpret28/1 -> o13/1
  Reinterpret27/1 -> o12/1
  Reinterpret26/1 -> o11/1
  Reinterpret25/1 -> o10/1
  Reinterpret24/1 -> o9/1
  Reinterpret23/1 -> o8/1
  Reinterpret22/1 -> o7/1
  Reinterpret21/1 -> o6/1
  Reinterpret20/1 -> o5/1
  Reinterpret19/1 -> o4/1
  Reinterpret18/1 -> o3/1
  Reinterpret17/1 -> o2/1
  Reinterpret16/1 -> o1/1
  Reinterpret15/1 -> Slice31/1, Slice15/1
  Reinterpret14/1 -> Slice30/1, Slice14/1
  Reinterpret13/1 -> Slice29/1, Slice13/1
  Reinterpret12/1 -> Slice28/1, Slice12/1
  Reinterpret11/1 -> Slice27/1, Slice11/1
  Reinterpret10/1 -> Slice26/1, Slice10/1
  Reinterpret9/1 -> Slice25/1, Slice9/1
  Reinterpret8/1 -> Slice24/1, Slice8/1
  Reinterpret7/1 -> Slice23/1, Slice7/1
  Reinterpret6/1 -> Slice22/1, Slice6/1
  Reinterpret5/1 -> Slice21/1, Slice5/1
  Reinterpret4/1 -> Slice20/1, Slice4/1
  Reinterpret3/1 -> Slice19/1, Slice3/1
  Reinterpret2/1 -> Slice18/1, Slice2/1
  Reinterpret1/1 -> Slice17/1, Slice1/1
  Reinterpret0/1 -> Slice16/1, Slice0/1
  Slice16/1 -> Concat0/1
  Slice0/1 -> Concat0/2
  Concat0/1 -> Reinterpret16/1
  i1/1 -> Reinterpret0/1
  Slice17/1 -> Concat1/1
  Slice1/1 -> Concat1/2
  Concat1/1 -> Reinterpret17/1
  i2/1 -> Reinterpret1/1
  Slice18/1 -> Concat2/1
  Slice2/1 -> Concat2/2
  Concat2/1 -> Reinterpret18/1
  i3/1 -> Reinterpret2/1
  Slice19/1 -> Concat3/1
  Slice3/1 -> Concat3/2
  Concat3/1 -> Reinterpret19/1
  i4/1 -> Reinterpret3/1
  Slice20/1 -> Concat4/1
  Slice4/1 -> Concat4/2
  Concat4/1 -> Reinterpret20/1
  i5/1 -> Reinterpret4/1
  Slice21/1 -> Concat5/1
  Slice5/1 -> Concat5/2
  Concat5/1 -> Reinterpret21/1
  i6/1 -> Reinterpret5/1
  Slice22/1 -> Concat6/1
  Slice6/1 -> Concat6/2
  Concat6/1 -> Reinterpret22/1
  i7/1 -> Reinterpret6/1
  Slice23/1 -> Concat7/1
  Slice7/1 -> Concat7/2
  Concat7/1 -> Reinterpret23/1
  i8/1 -> Reinterpret7/1
  Slice24/1 -> Concat8/1
  Slice8/1 -> Concat8/2
  Concat8/1 -> Reinterpret24/1
  i9/1 -> Reinterpret8/1
  Slice25/1 -> Concat9/1
  Slice9/1 -> Concat9/2
  Concat9/1 -> Reinterpret25/1
  i10/1 -> Reinterpret9/1
  Slice26/1 -> Concat10/1
  Slice10/1 -> Concat10/2
  Concat10/1 -> Reinterpret26/1
  i11/1 -> Reinterpret10/1
  Slice27/1 -> Concat11/1
  Slice11/1 -> Concat11/2
  Concat11/1 -> Reinterpret27/1
  i12/1 -> Reinterpret11/1
  Slice28/1 -> Concat12/1
  Slice12/1 -> Concat12/2
  Concat12/1 -> Reinterpret28/1
  i13/1 -> Reinterpret12/1
  Slice29/1 -> Concat13/1
  Slice13/1 -> Concat13/2
  Concat13/1 -> Reinterpret29/1
  i14/1 -> Reinterpret13/1
  Slice30/1 -> Concat14/1
  Slice14/1 -> Concat14/2
  Concat14/1 -> Reinterpret30/1
  i15/1 -> Reinterpret14/1
  Slice31/1 -> Concat15/1
  Slice15/1 -> Concat15/2
  Concat15/1 -> Reinterpret31/1
  i16/1 -> Reinterpret15/1

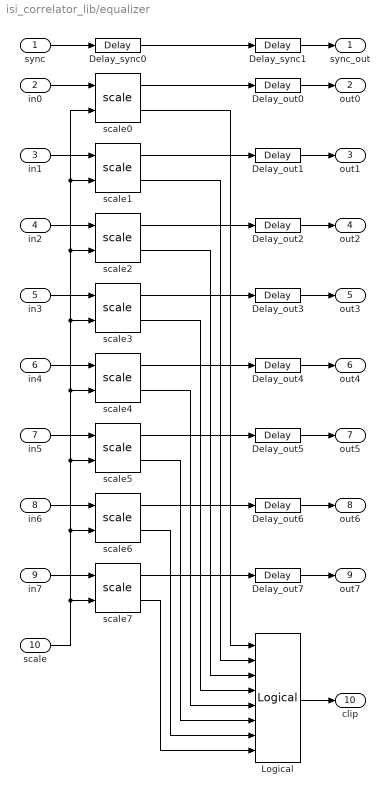
== system isi_correlator_lib/equalizer ==
  sync : Inport
  in0 : Inport  Port=2
  in1 : Inport  Port=3
  in2 : Inport  Port=4
  in3 : Inport  Port=5
  in4 : Inport  Port=6
  in5 : Inport  Port=7
  in6 : Inport  Port=8
  in7 : Inport  Port=9
  scale : Inport  Port=10
  Delay_out{0..7} (8 alike) : xbsIndex_r4/Delay  en=off  latency=3  dbl_ovrd=off  reg_retiming=off  block_type=delay
  Delay_sync0 : xbsIndex_r4/Delay  en=off  latency=5  dbl_ovrd=off  reg_retiming=off  block_type=delay
  Delay_sync1 : xbsIndex_r4/Delay  en=off  latency=3  dbl_ovrd=off  reg_retiming=off  block_type=delay
  Logical : xbsIndex_r4/Logical  logical_function=OR  inputs=8  en=off  latency=3  precision=Full  arith_type=Unsigned  n_bits=16  bin_pt=0  align_bp=on  dbl_ovrd=off  block_type=logical
  scale{0..7} (8 alike) : isi_correlator_lib/scale  SystemSampleTime=-1  in_bit_width=in_bit_width  in_bin_point=in_bin_point  coeff_bit_width=coeff_bit_width  coeff_bin_point=coeff_bin_point  out_bit_width=out_bit_width  out_bin_point=out_bin_point
  sync_out : Outport
  out0 : Outport  Port=2
  out1 : Outport  Port=3
  out2 : Outport  Port=4
  out3 : Outport  Port=5
  out4 : Outport  Port=6
  out5 : Outport  Port=7
  out6 : Outport  Port=8
  out7 : Outport  Port=9
  clip : Outport  Port=10
  wires:
  in0/1 -> scale0/1
  in1/1 -> scale1/1
  in2/1 -> scale2/1
  in3/1 -> scale3/1
  in4/1 -> scale4/1
  in5/1 -> scale5/1
  in6/1 -> scale6/1
  in7/1 -> scale7/1
  scale0/1 -> Delay_out0/1
  scale1/1 -> Delay_out1/1
  scale2/1 -> Delay_out2/1
  scale3/1 -> Delay_out3/1
  scale4/1 -> Delay_out4/1
  scale5/1 -> Delay_out5/1
  scale6/1 -> Delay_out6/1
  scale7/1 -> Delay_out7/1
  scale7/2 -> Logical/8
  scale6/2 -> Logical/7
  scale5/2 -> Logical/6
  scale4/2 -> Logical/5
  scale3/2 -> Logical/4
  scale2/2 -> Logical/3
  scale1/2 -> Logical/2
  scale0/2 -> Logical/1
  Delay_sync0/1 -> Delay_sync1/1
  Delay_sync1/1 -> sync_out/1
  sync/1 -> Delay_sync0/1
  Logical/1 -> clip/1
  scale/1 -> scale0/2, scale1/2, scale2/2, scale3/2, scale4/2, scale5/2, scale6/2, scale7/2
  Delay_out0/1 -> out0/1
  Delay_out1/1 -> out1/1
  Delay_out2/1 -> out2/1
  Delay_out3/1 -> out3/1
  Delay_out4/1 -> out4/1
  Delay_out5/1 -> out5/1
  Delay_out6/1 -> out6/1
  Delay_out7/1 -> out7/1

== system isi_correlator_lib/fake_xaui ==
  sync : Inport  OutDataType=sfix(16)  OutScaling=2^0
  data_fifo_in : Inport  Port=2  OutDataType=sfix(16)  OutScaling=2^0
  valid_fifo_in : Inport  Port=3  OutDataType=sfix(16)  OutScaling=2^0
  Delay1 : xbsIndex_r4/Delay  en=off  latency=latency  dbl_ovrd=off  reg_retiming=off  block_type=delay
  Delay2 : xbsIndex_r4/Delay  en=off  latency=latency  dbl_ovrd=off  reg_retiming=off  block_type=delay
  Delay3 : xbsIndex_r4/Delay  en=off  latency=latency  dbl_ovrd=off  reg_retiming=off  block_type=delay
  sync_out : Outport  OutDataType=sfix(16)  OutScaling=2^0
  data_fifo : Outport  Port=2  OutDataType=sfix(16)  OutScaling=2^0
  valid_fifo : Outport  Port=3  OutDataType=sfix(16)  OutScaling=2^0
  wires:
  Delay3/1 -> valid_fifo/1
  Delay2/1 -> data_fifo/1
  Delay1/1 -> sync_out/1
  sync/1 -> Delay1/1
  data_fifo_in/1 -> Delay2/1
  valid_fifo_in/1 -> Delay3/1

== system isi_correlator_lib/pulse_hold ==
  din : Inport  OutDataType=sfix(16)  OutScaling=2^0
  rst : Inport  Port=2  OutDataType=sfix(16)  OutScaling=2^0
  Register : xbsIndex_r4/Register  init=0  rst=on  en=on  dbl_ovrd=off  block_type=register
  hold : Outport  OutDataType=sfix(16)  OutScaling=2^0
  wires:
  din/1 -> Register/1, Register/3
  rst/1 -> Register/2
  Register/1 -> hold/1
